simulink model "Miscellaneous_Unit"  (R2018a)
settings: Solver=ode2  StartTime=0.0  StopTime=inf  FixedStep=0.002  RelTol=1e-3  EnableMultiTasking=on
libraries: simulink x2, quarc_library x1
settings Model: Creator=User  LastModifiedBy=User
settings SolverCC: PositivePriorityOrder=on
settings RTWCC: SystemTargetFile=quarc_linux_nvidia.tlc  TemplateMakefile=quarc_linux_nvidia_tmf  Description=QUARC Linux Nvidia Target
settings STFCustomTargetCC: TargetLibSuffix=.a  TargetPreCompLibLocation=C:\PROGRA~3\QUARC\lib\2018a\LINUX_~1\release  TargetLangStandard=C99 (ISO)  ConcurrentExecutionCompliant=on  SystemTargetFile=quarc_linux_nvidia.tlc
settings GRTTargetCC: TargetLibSuffix=.a  TargetPreCompLibLocation=C:\PROGRA~3\QUARC\lib\2018a\LINUX_~1\release  ParMdlRefBuildCompliant=off  CompOptLevelCompliant=off  CombineOutputUpdateFcns=off  MatFileLogging=off  CPPClassGenCompliant=off  GRTInterface=on  UseToolchainInfoCompliant=off  ExtMode=on  ExtModeMexFile=quarc_comm  ExtModeMexArgs='-w -d /tmp -uri %u'

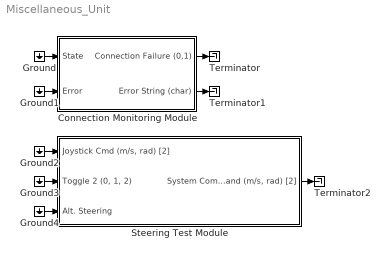
== system Miscellaneous_Unit ==
  Connection Monitoring Module : Subsystem
  Ground{,1..4} (5 alike) : Ground
  Steering Test Module : Subsystem
  Terminator : Terminator
  Terminator1 : Terminator
  Terminator2 : Terminator
  wires:
  Ground1/1 -> Connection Monitoring Module/2(Error)
  Connection Monitoring Module/2(Error String (char)) -> Terminator1/1
  Connection Monitoring Module/1(Connection Failure (0,1)) -> Terminator/1
  Ground3/1 -> Steering Test Module/2("Toggle 2 (0, 1, 2)")
  Steering Test Module/1("System Command (m/s, rad) [2]") -> Terminator2/1
  Ground2/1 -> Steering Test Module/1("Joystick Cmd (m/s, rad) [2]")
  Ground/1 -> Connection Monitoring Module/1(State)
  Ground4/1 -> Steering Test Module/3(Alt. Steering)

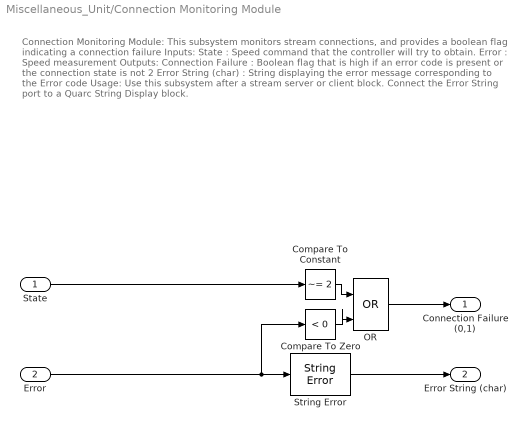
== system Miscellaneous_Unit/Connection Monitoring Module ==
  note: Connection Monitoring Module:
      |
      | This subsystem monitors stream connections, and provides a boolean flag indicating a connection failure
      |
      | Inputs:
      | State : Speed command that the controller will try to obtain.
      | Error : Speed measurement
      |
      | Outputs:
      | Connection Failure : Boolean flag that is high if an error code is present or the connection state is not 2
      | Error String (char) : String displaying the error message corresponding to the Error code
      |
      | Usage:
      | Use this subsystem after a stream server or client block. Connect the Error String port to a Quarc String Display block.
  State : Inport
  Error : Inport  Port=2
  Compare To Constant : simulink/Logic and Bit Operations/Compare To Constant  relop=~=  const=2  OutDataTypeStr=boolean
  Compare To Zero : simulink/Logic and Bit Operations/Compare To Zero  relop=<  OutDataTypeStr=boolean
  OR : Logic  Operator=OR  IconShape=distinctive  AllPortsSameDT=off  OutDataTypeStr=boolean
  String Error : quarc_library/Strings/String Error  default_string=No error occurred.  max_length=512  variable_size=off
      settings: SourceProductName=QUARC Targets
  Connection Failure (0,1) : Outport
  Error String (char) : Outport  Port=2
  wires:
  Error/1 -> Compare To Zero/1, String Error/1
  Compare To Constant/1 -> OR/1
  String Error/1 -> Error String (char)/1
  State/1 -> Compare To Constant/1
  Compare To Zero/1 -> OR/2
  OR/1 -> Connection Failure (0,1)/1

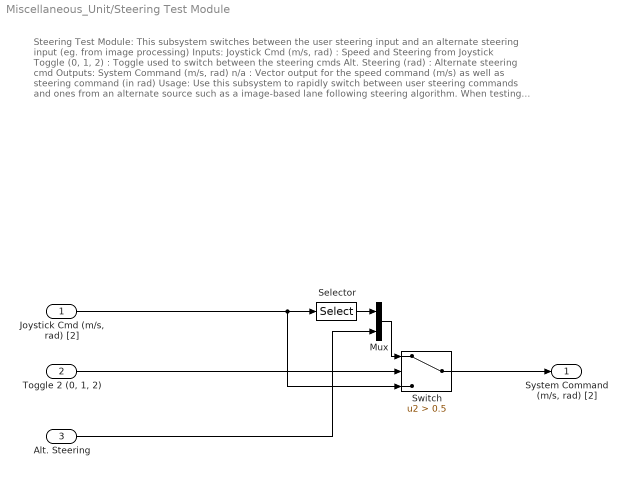
== system Miscellaneous_Unit/Steering Test Module ==
  note: Steering Test Module:
      |
      | This subsystem switches between the user steering input and an alternate steering input (eg. from image processing)
      |
      | Inputs:
      | Joystick Cmd (m/s, rad) : Speed and Steering from Joystick
      | Toggle (0, 1, 2) : Toggle used to switch between the steering cmds
      | Alt. Steering (rad) : Alternate steering cmd
      |
      | Outputs:
      | System Command (m/s, rad) n/a : Vector output for the speed command (m/s) as well as steering command (in rad)
      |
      | Usage:
      | Use this subsystem to rapidly switch between user steering commands and ones from an alternate source such as a image-based lane following steering algorithm. When testing the algorithm, the user may need to override the steering to prevent crashes.
  "Joystick Cmd (m/s, rad) [2]" : Inport
  "Toggle 2 (0, 1, 2)" : Inport  Port=2
  Alt. Steering : Inport  Port=3
  Mux : Mux  Inputs=2
  Selector : Selector  InputPortWidth=2  IndexOptions=Index vector (dialog)  Indices=[1]  OutputSizes=1
  Switch : Switch  Criteria=u2 > Threshold  Threshold=0.5
  "System Command (m/s, rad) [2]" : Outport
  wires:
  Switch/1 -> "System Command (m/s, rad) [2]"/1
  Selector/1 -> Mux/1
  Alt. Steering/1 -> Mux/2
  "Joystick Cmd (m/s, rad) [2]"/1 -> Switch/3, Selector/1
  Mux/1 -> Switch/1
  "Toggle 2 (0, 1, 2)"/1 -> Switch/2
